simulink model "mcp3008_task"  (Simulink 3.00)
undefined symbols (not defined in the file): y2
libraries: mathlib x11, paramlib x8, arclib x2, speclib x1

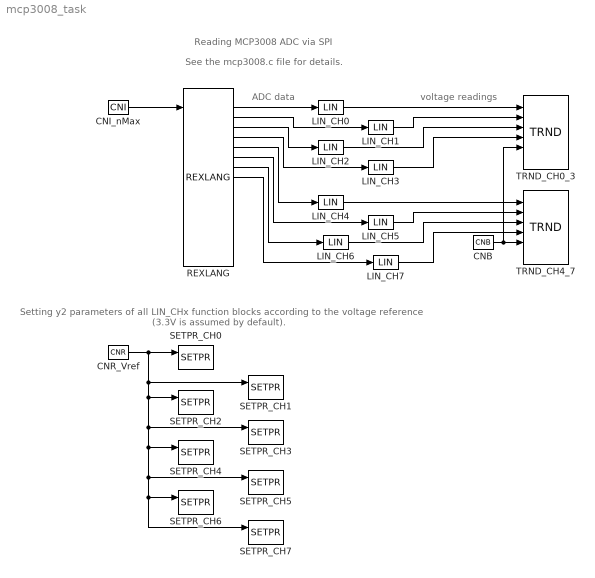
== system mcp3008_task ==
  note: Reading MCP3008 ADC via SPI
  note: See the mcp3008.c file for details.
  note: ADC data
  note: voltage readings
  note: Setting y2 parameters of all LIN_CHx function blocks
      | according to the voltage reference (3.3V is assumed
      | by default).
  CNB : mathlib/CNB  YCN=on
  CNI_nMax : mathlib/CNI  icn=7
  CNR_Vref : mathlib/CNR  ycn=3.3
  LIN_CH{0..1,3,5..7} (6 alike) : mathlib/LIN  u1=0  y1=0  u2=1023  y2=3.3
  LIN_CH2 : mathlib/LIN  u1=1023  y1=0  u2=1048575  y2=3.3
  LIN_CH4 : mathlib/LIN  u1=1023  y1=0  u2=1048575  y2=3.3
  REXLANG : speclib/REXLANG  SystemSampleTime=-1  tab_matlab=BASIC  srcname=mcp3008.c  srctype=1: STL  stack=0  debug=1: No check  p0=0  p1=0  p2=0  p3=0  p4=0  p5=0  p6=0  p7=0  p8=0  p9=0  p10=0  p11=0  p12=0  p13=0  p14=0  p15=0  fname=/dev/spidev0.0
  SETPR_CH0 : paramlib/SETPR  sc=.LIN_CH0:y2  SETF=off
  SETPR_CH1 : paramlib/SETPR  sc=.LIN_CH1:y2  SETF=off
  SETPR_CH2 : paramlib/SETPR  sc=.LIN_CH2:y2  SETF=off
  SETPR_CH3 : paramlib/SETPR  sc=.LIN_CH3:y2  SETF=off
  SETPR_CH4 : paramlib/SETPR  sc=.LIN_CH4:y2  SETF=off
  SETPR_CH5 : paramlib/SETPR  sc=.LIN_CH5:y2  SETF=off
  SETPR_CH6 : paramlib/SETPR  sc=.LIN_CH6:y2  SETF=off
  SETPR_CH7 : paramlib/SETPR  sc=.LIN_CH7:y2  SETF=off
  TRND_CH0_3 : arclib/TRND  n=4  l=1000  btype=8: Double  ptype1=1: Store  ptype2=1: Store  ptype3=1: Store  ptype4=1: Store  pfac=1  afac=0  arc=0  id=1  Title=Channels 0..3
  TRND_CH4_7 : arclib/TRND  n=4  l=1000  btype=8: Double  ptype1=1: Store  ptype2=1: Store  ptype3=1: Store  ptype4=1: Store  pfac=1  afac=0  arc=0  id=2  Title=Channels 4..7
  wires:
  CNB/1 -> TRND_CH4_7/5, TRND_CH0_3/5
  CNI_nMax/1 -> REXLANG/2
  CNR_Vref/1 -> SETPR_CH0/1, SETPR_CH1/1, SETPR_CH2/1, SETPR_CH3/1, SETPR_CH4/1, SETPR_CH5/1, SETPR_CH6/1, SETPR_CH7/1
  LIN_CH0/1 -> TRND_CH0_3/1
  LIN_CH1/1 -> TRND_CH0_3/2
  LIN_CH2/1 -> TRND_CH0_3/3
  LIN_CH3/1 -> TRND_CH0_3/4
  LIN_CH4/1 -> TRND_CH4_7/1
  LIN_CH5/1 -> TRND_CH4_7/2
  LIN_CH6/1 -> TRND_CH4_7/3
  LIN_CH7/1 -> TRND_CH4_7/4
  REXLANG/2 -> LIN_CH0/1
  REXLANG/3 -> LIN_CH1/1
  REXLANG/4 -> LIN_CH2/1
  REXLANG/5 -> LIN_CH3/1
  REXLANG/6 -> LIN_CH4/1
  REXLANG/7 -> LIN_CH5/1
  REXLANG/8 -> LIN_CH6/1
  REXLANG/9 -> LIN_CH7/1
